simulink model "Linearni_system"  (R2020a)
settings: Solver=FixedStepAuto  StartTime=0.0  StopTime=50  FixedStep=0.01  RelTol=1e-3
values from neighbouring files (symbols this model uses):
  dphi = 0    [Model_kyvadla_na_voziku_m.m]
  dx = 0    [Model_kyvadla_na_voziku_m.m]
  f = 0    [Model_kyvadla_na_voziku_m.m]
  g = 9.81    [Model_kyvadla_na_voziku_m.m]
  l = 1    [Model_kyvadla_na_voziku_m.m]
  phi = deg2rad(5)    [Model_kyvadla_na_voziku_m.m]
  sys = ss(A, B, C, D)    [Model_kyvadla_na_voziku_m.m]
  x = 0    [Model_kyvadla_na_voziku_m.m]
settings Model: Creator=Jiří  LastModifiedBy=Jiří
settings SolverCC: AlgebraicLoopSolver=LineSearch

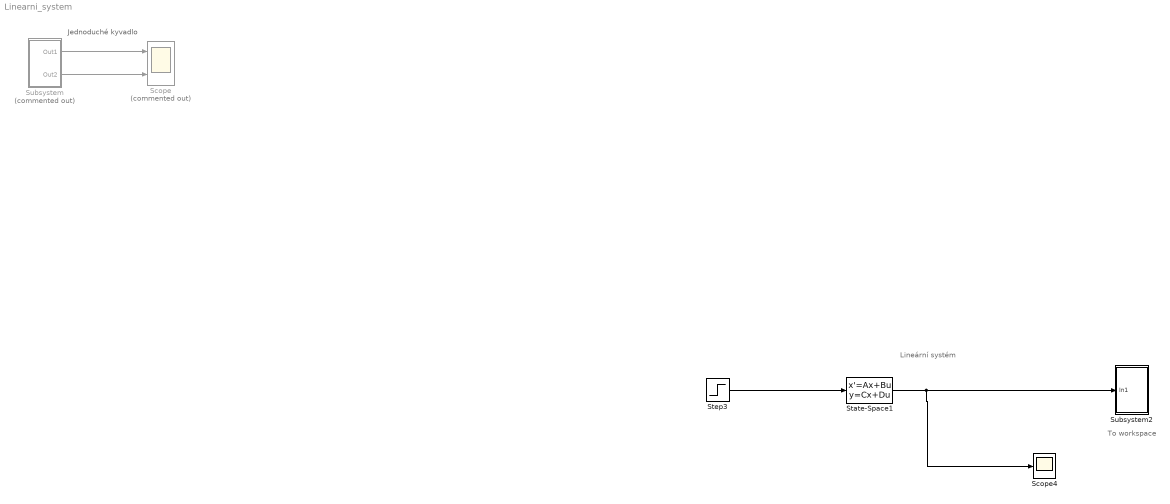
== system Linearni_system ==
  note: Lineární systém
  note: Jednoduché kyvadlo
  note: To workspace
  Scope : Scope  Commented=on  NumInputPorts=2
  Scope4 : Scope
  State-Space1 : StateSpace  A=sys.A  B=sys.B  C=sys.C  D=sys.D  InitialCondition=[x, phi, dx, dphi]
  Step3 : Step  Time=10  After=f  SampleTime=1
  Subsystem : Subsystem  Commented=on
  Subsystem2 : Subsystem
  wires:
  Subsystem/1(Out1) -> Scope/1
  Subsystem/2(Out2) -> Scope/2
  State-Space1/1 -> Scope4/1, Subsystem2/1(In1)
  Step3/1 -> State-Space1/1

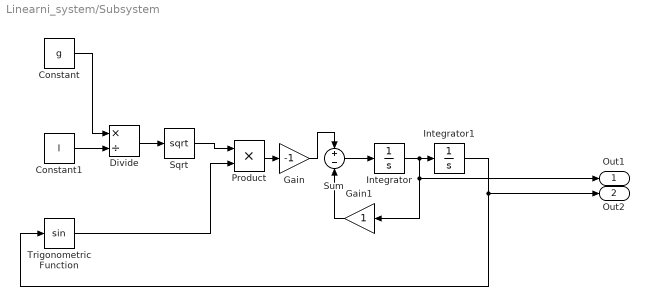
== system Linearni_system/Subsystem ==
  Constant : Constant  Value=g
  Constant1 : Constant  Value=l
  Divide : Product  Inputs=*/
  Gain : Gain  Gain=-1
  Gain1 : Gain
  Integrator : Integrator
  Integrator1 : Integrator  InitialCondition=1
  Product : Product
  Sqrt : Sqrt  SaturateOnIntegerOverflow=on
  Sum : Sum  Inputs=+-
  Trigonometric Function : Trigonometry
  Out1 : Outport
  Out2 : Outport  Port=2
  wires:
  Integrator/1 -> Gain1/1, Out1/1, Integrator1/1
  Constant/1 -> Divide/1
  Trigonometric Function/1 -> Product/2
  Divide/1 -> Sqrt/1
  Product/1 -> Gain/1
  Constant1/1 -> Divide/2
  Integrator1/1 -> Out2/1, Trigonometric Function/1
  Sqrt/1 -> Product/1
  Gain/1 -> Sum/1
  Sum/1 -> Integrator/1
  Gain1/1 -> Sum/2

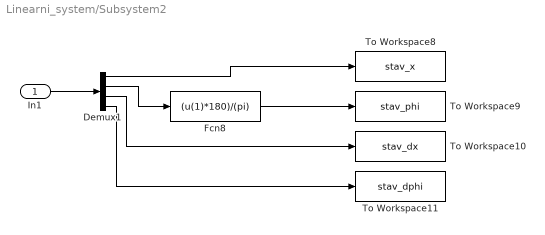
== system Linearni_system/Subsystem2 ==
  In1 : Inport
  Demux1 : Demux
  Fcn8 : Fcn  Expr=(u(1)*180)/(pi)
  To Workspace10 : ToWorkspace  VariableName=stav_dx  SaveFormat=Timeseries  SampleTime=-1
  To Workspace11 : ToWorkspace  VariableName=stav_dphi  SaveFormat=Timeseries  SampleTime=-1
  To Workspace8 : ToWorkspace  VariableName=stav_x  SaveFormat=Timeseries  SampleTime=-1
  To Workspace9 : ToWorkspace  VariableName=stav_phi  SaveFormat=Timeseries  SampleTime=-1
  wires:
  Demux1/3 -> To Workspace10/1
  Fcn8/1 -> To Workspace9/1
  Demux1/4 -> To Workspace11/1
  Demux1/1 -> To Workspace8/1
  In1/1 -> Demux1/1
  Demux1/2 -> Fcn8/1
